simulink model "Modello_Simulink"  (R2020b)
settings: Solver=ode4  StartTime=0.0  StopTime=10  FixedStep=0.05  RelTol=1e-3
values from neighbouring files (symbols this model uses):
  EQ_POS = [pi,0]    [init.m]
  INITIAL_CONDITIONS = [0,0,0,0]    [Alternative_Init.m]    (also in init.m = [pi,0,0,0]; lqr_init.m = [pi + pi/12, -pi/12, 0, 0])
  K_d = -K(3:4)    [DaCBarF.m]    (also in Pendubot_init.m; Segway_paper.m = 0.1; init.m = K(:,3:4); lqr_init.m)
  K_p = -K(1:2)    [DaCBarF.m]    (also in Pendubot_init.m; Segway_paper.m = 1; init.m = K(:,1:2); lqr_init.m)
  PARAM = [m1,m2,I1,lc1,l2,lc2,I1,I2]    [Alternative_Init.m]    (also in init.m)
  tau_eq = mp*G*l*sin(thetae)    [Cartpole.m]    (also in DaCBarF.m = a4*sin(Q1E)+a5*sin(Q1E+Q2E); Pendubot_init.m = a4*sin(q1e)+a5*sin(q1e+q2e); init.m = a4*sin(q1e) + a5*sin(q1e+q2e); lqr_init.m = [a4*sin(q1e)+a5*sin(q1e+q2e)])
settings Model: Creator=gianl  LastModifiedBy=loren
settings DataIOCC: ReturnWorkspaceOutputs=off

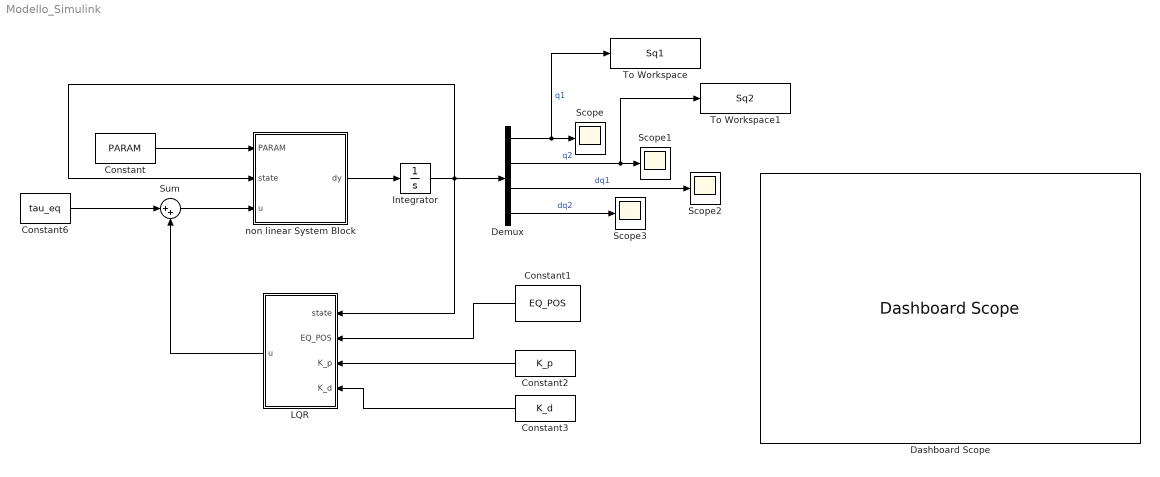
== system Modello_Simulink ==
  Constant : Constant  Value=PARAM
  Constant1 : Constant  Value=EQ_POS
  Constant2 : Constant  Value=K_p
  Constant3 : Constant  Value=K_d
  Constant6 : Constant  Value=tau_eq
  Dashboard Scope : DashboardScope
  Demux : Demux
  Integrator : Integrator  InitialCondition=INITIAL_CONDITIONS
  LQR : MATLAB Function  TreatAsAtomicUnit=on
  Scope{,1..3} (4 alike) : Scope
  Sum : Sum  Inputs=|++
  To Workspace : ToWorkspace  VariableName=Sq1  SaveFormat=Timeseries  SampleTime=-1
  To Workspace1 : ToWorkspace  VariableName=Sq2  SaveFormat=Timeseries  SampleTime=-1
  non linear System Block : MATLAB Function  TreatAsAtomicUnit=on
  wires:
  Constant/1 -> non linear System Block/1(PARAM)
  non linear System Block/1(dy) -> Integrator/1
  Integrator/1 -> non linear System Block/2(state), Demux/1, LQR/1(state)
  LQR/1(u) -> Sum/2
  Constant2/1 -> LQR/3(K_p)
  Constant1/1 -> LQR/2(EQ_POS)
  Demux/1 -> To Workspace/1, Scope/1  "q1"
  Demux/2 -> To Workspace1/1, Scope1/1  "q2"
  Demux/3 -> Scope2/1  "dq1"
  Demux/4 -> Scope3/1  "dq2"
  Constant3/1 -> LQR/4(K_d)
  Sum/1 -> non linear System Block/3(u)
  Constant6/1 -> Sum/1

== matlab function Modello_Simulink/LQR ==
  data: state input size=4; EQ_POS input size=2; u output size=2; K_p input size=[1,2]; K_d input size=[1,2]
function u = controller(state, EQ_POS, K_p, K_d)
   
    q1 = state(1);
    q2 = state(2);
    dq1 = state(3);
    dq2 = state(4);
    q1e = EQ_POS(1);
    q2e = EQ_POS(2);
    
    q = [q1; q2];
    q_dot = [dq1; dq2];
    qe = [q1e; q2e];

tau = K_p*(q-qe) + K_d*q_dot;

u=[tau,0]';
end

== matlab function Modello_Simulink/non linear System Block ==
  data: PARAM input; state input; u input size=2; dy output size=4
function dy = nonlinearSys(PARAM,state,u)
m1 = PARAM(1);              % giunto 1 mass
m2 = PARAM(2);              % giunto 2 mass
l1 = PARAM(3);          % lunghezza primo giunto
lc1 = PARAM(4);          % centro di massa giunto 1
l2 = PARAM(5);
lc2 = PARAM(6);
I1 = PARAM(7);
I2 = PARAM(8);
g= 9.81;

q1 = state(1);
q2 = state(2);
dq1 = state(3);
dq2= state(4);

a1 = I1+ I2+ m1*lc1^2+m2*(l1^2+lc2^2);
a2 = m2*l1*lc2;
a3 = I2 + m2*lc2^2;
a4 = g*(m1*lc1+m2*l1);
a5 = g*m2*lc2;

M = [a1+2*a2*cos(q2), a3+a2*cos(q2);
     a3+a2*cos(q2), a3];

c = [a2*dq2*(dq2+2*dq1)*sin(q2);
    a2*dq1^2*sin(q2)];
e = [ a4*sin(q1) + a5*sin(q1+q2);
    a5*sin(q1+q2)];
n = c+e;

f = [dq1;
    dq2;
    -inv(M)*n;
   ];

g =[0,0;
    0,0;
    inv(M);
    ];
dy =f+g*u;
